simulink model "myproject_exec"  (Simulink 3.00)
libraries: execlib x5

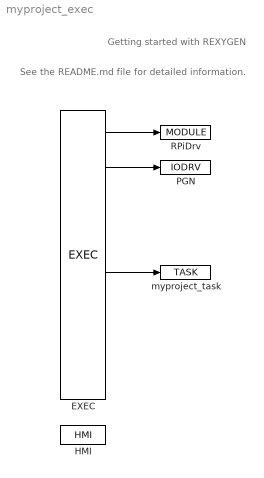
== system myproject_exec ==
  note: See the README.md file for
      | detailed information.
  note: Getting started with REXYGEN
  EXEC : execlib/EXEC  target=Generic target device  tick=0.05  ntick0=2  ntick1=50  ntick2=100  ntick3=1200  pri0=5  pri1=9  pri2=13  pri3=18
  HMI : execlib/HMI  IncludeHMI=on  HmiDir=hmi  SourceDir=hmisrc  GenerateWebWatch=off  GenerateRexHMI=on  RedirectToHMI=on  Compression=off
  PGN : execlib/IODRV  module=RPiDrv  classname=PgnDrv  factor=1  stack=10240  pri=3  timer=off
  RPiDrv : execlib/MODULE
  myproject_task : execlib/TASK  factor=1  start=0  stop=1  stack=10240  MDLOPEN=on
  wires:
  EXEC/1 -> RPiDrv/1
  EXEC/2 -> PGN/1
  EXEC/5 -> myproject_task/1
